simulink model "linear_trajectory_planning"  (R2023a)
settings: configuration reference "config" (kept outside this file)
model workspace (MAT data in the model file):
  enc_line_inv_p_n = Simulink.Parameter
  enc_line_inv_p_n.Value = 0.0001
  enc_line_inv_p_n.Description = '编码器分辨率 倒数   
    | '
  enc_line_inv_p_n.DataType = 'single'
  enc_line_inv_p_n.Complexity = 'real'
  enc_line_inv_p_n.Dimensions = [1 1]
  init_flag = Simulink.Signal
  init_flag.Description = '初始化信号  0  1 需要被初始化'
  init_flag.DataType = 'uint8'
  init_flag.Dimensions = 1
  init_flag.DimensionsMode = 'auto'
  init_flag.Complexity = 'auto'
  init_flag.SampleTime = -1
  init_flag.SamplingMode = 'auto'
  kFs = Simulink.Parameter
  kFs.Value = 10000
  kFs.Description = '位置环 速度环执行频率  仅用于仿真'
  kFs.DataType = 'double'
  kFs.Complexity = 'real'
  kFs.Dimensions = [1 1]
  tp = Simulink.Parameter
  tp.Value = 0.0001
  tp.Description = '位置环速度环执行周期  s'
  tp.DataType = 'single'
  tp.Complexity = 'real'
  tp.Dimensions = [1 1]
  wn_Hz = Simulink.Parameter
  wn_Hz.Value = 400
  wn_Hz.Description = '速度观测器带宽 Hz'
  wn_Hz.DataType = 'single'
  wn_Hz.Complexity = 'real'
  wn_Hz.Dimensions = [1 1]
settings Model: DataDictionary=model_config.sldd  ParameterArgumentNames=enc_line_inv_p_n,tp,wn_Hz  Creator=huangcheng  LastModifiedBy=Administrator
settings ConfigSetRef: SourceName=config

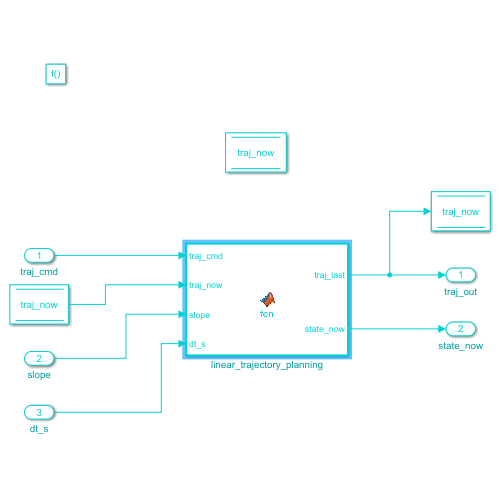
[thumbnail: Simulink's stored preview of the top-level diagram]
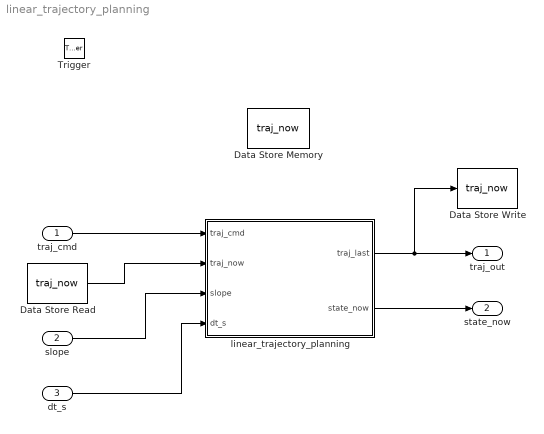
== system linear_trajectory_planning ==
  traj_cmd : Inport  OutDataTypeStr=single
  slope : Inport  Port=2  OutDataTypeStr=single
  dt_s : Inport  Port=3  OutDataTypeStr=single
  Trigger : TriggerPort  TriggerType=function-call  VariantControl=(inherit)  PortDimensions=1
  Data Store Memory : DataStoreMemory  DataStoreName=traj_now  WriteAfterWriteMsg=warning  ShowAdditionalParam=off  OutDataTypeStr=single
  Data Store Read : DataStoreRead  DataStoreName=traj_now  IndexOptions=Index vector (dialog)  Indices=1  OutputSizes=1
  Data Store Write : DataStoreWrite  DataStoreName=traj_now  IndexOptions=Index vector (dialog)  Indices=1  OutputSizes=1
  linear_trajectory_planning : MATLAB Function  TreatAsAtomicUnit=on
  traj_out : Outport  OutDataTypeStr=single
  state_now : Outport  Port=2  OutDataTypeStr=int8
  wires:
  traj_cmd/1 -> linear_trajectory_planning/1(traj_cmd)
  Data Store Read/1 -> linear_trajectory_planning/2(traj_now)
  slope/1 -> linear_trajectory_planning/3(slope)
  dt_s/1 -> linear_trajectory_planning/4(dt_s)
  linear_trajectory_planning/1(traj_last) -> traj_out/1, Data Store Write/1
  linear_trajectory_planning/2(state_now) -> state_now/1

== matlab function linear_trajectory_planning/linear_trajectory_planning ==
  data: traj_cmd input; traj_last output; traj_now input; slope input; dt_s input; state_now output
function [traj_last, state_now] = fcn(traj_cmd, traj_now, slope, dt_s)
 
% state_now  规划状态  
% 0 初始状态
% 1 规划完成
% 2 规划中

traj_last_temp = single(0);
state_now_temp = int8(0);

if traj_now > traj_cmd
    traj_last_temp = traj_now - slope * dt_s;
    state_now_temp = int8(2);
    if traj_last_temp < traj_cmd
        traj_last_temp = traj_cmd;
        state_now_temp = int8(1);
    end
else
    traj_last_temp = traj_now + slope * dt_s;
    state_now_temp = int8(2);
    if traj_last_temp > traj_cmd
        traj_last_temp = traj_cmd;
        state_now_temp = int8(1);
    end

end

traj_last = traj_last_temp;
state_now = state_now_temp;
